simulink model "ActuatorModels_alpha"  (R2017a)
settings: Solver=VariableStepAuto  StartTime=0.0  StopTime=10.0  RelTol=1e-3
undefined symbols (not defined in the file or in its folder): fin_max, fin_maxrate, fin_min, omega, wn_fin, z_fin, zeta
libraries: aerolibactuator x2
settings Model: Creator=AHKh  LastModifiedBy=AHKh

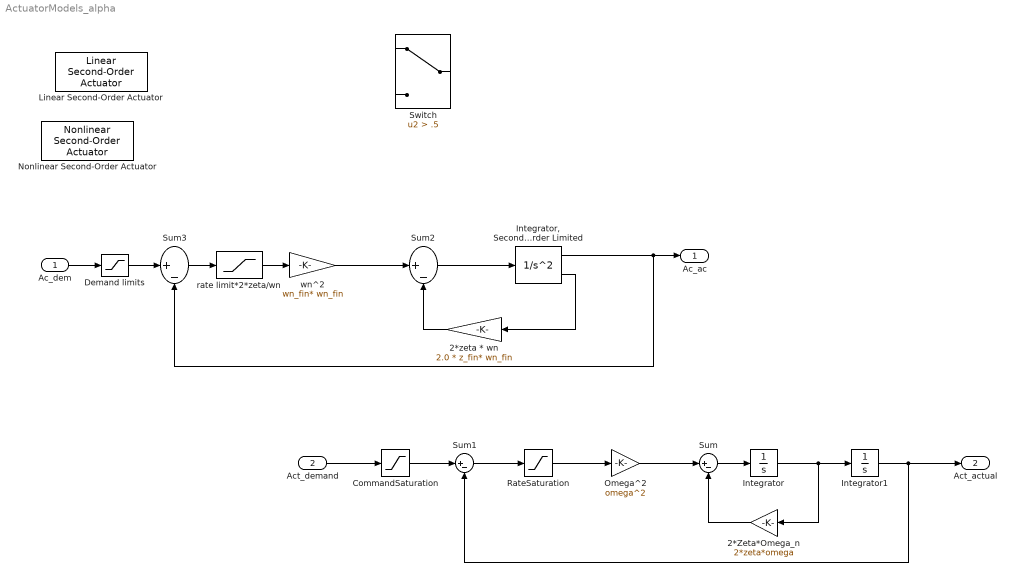
== system ActuatorModels_alpha ==
  Ac_dem : Inport
  Act_demand : Inport  Port=2
  2*Zeta*Omega_n : Gain  Gain=2*zeta*omega
  2*zeta * wn : Gain  Gain=2.0 * z_fin* wn_fin  SaturateOnIntegerOverflow=on  OutDataTypeStr=Inherit: Same as input  ParamDataTypeStr=Inherit: Same as input
  CommandSaturation : Saturate
  Demand limits : Saturate  UpperLimit=fin_max  LowerLimit=fin_min
  Integrator : Integrator
  "Integrator, Second-Order Limited" : SecondOrderIntegrator  ICX=fin_act_0  LimitX=on  UpperLimitX=fin_max  LowerLimitX=fin_min  ICDXDT=fin_act_vel  LimitDXDT=on  UpperLimitDXDT=fin_maxrate  LowerLimitDXDT=-fin_maxrate
  Integrator1 : Integrator
  Linear Second-Order Actuator : aerolibactuator/Linear Second-Order Actuator  wn_fin=1  z_fin=0.3  fin_act_0=0  fin_act_vel=0
      settings: SourceProductName=Aerospace Blockset  SourceProductBaseCode=AE
  Nonlinear Second-Order Actuator : aerolibactuator/Nonlinear Second-Order Actuator  wn_fin=1  z_fin=0.3  fin_max=20*pi/180  fin_min=-20*pi/180  fin_maxrate=500*pi/180  fin_act_0=0  fin_act_vel=0
      settings: SourceProductName=Aerospace Blockset  SourceProductBaseCode=AE
  Omega^2 : Gain  Gain=omega^2
  RateSaturation : Saturate
  Sum : Sum  Inputs=|+-
  Sum1 : Sum  Inputs=|+-
  Sum2 : Sum  Inputs=|+-  SaturateOnIntegerOverflow=on  InputSameDT=on  OutDataTypeStr=Inherit: Same as first input
  Sum3 : Sum  Inputs=|+-  SaturateOnIntegerOverflow=on  InputSameDT=on  OutDataTypeStr=Inherit: Same as first input
  Switch : Switch  Criteria=u2 > Threshold  Threshold=.5
  rate limit*2*zeta/wn : Saturate  UpperLimit=fin_maxrate*2*z_fin/wn_fin  LowerLimit=-fin_maxrate*2*z_fin/wn_fin
  wn^2 : Gain  Gain=wn_fin* wn_fin  SaturateOnIntegerOverflow=on  OutDataTypeStr=Inherit: Same as input  ParamDataTypeStr=Inherit: Same as input
  Ac_ac : Outport  InitialOutput=0
  Act_actual : Outport  Port=2
  wires:
  wn^2/1 -> Sum2/1
  "Integrator, Second-Order Limited"/2 -> 2*zeta * wn/1
  Sum3/1 -> rate limit*2*zeta/wn/1
  Sum2/1 -> "Integrator, Second-Order Limited"/1
  Ac_dem/1 -> Demand limits/1
  Demand limits/1 -> Sum3/1
  2*zeta * wn/1 -> Sum2/2
  "Integrator, Second-Order Limited"/1 -> Sum3/2, Ac_ac/1
  rate limit*2*zeta/wn/1 -> wn^2/1
  Integrator/1 -> 2*Zeta*Omega_n/1, Integrator1/1
  2*Zeta*Omega_n/1 -> Sum/2
  Sum/1 -> Integrator/1
  Omega^2/1 -> Sum/1
  RateSaturation/1 -> Omega^2/1
  Sum1/1 -> RateSaturation/1
  Integrator1/1 -> Sum1/2, Act_actual/1
  CommandSaturation/1 -> Sum1/1
  Act_demand/1 -> CommandSaturation/1
